simulink model "PenduloSimple"  (R2016a)
settings: Solver=VariableStepAuto  StartTime=0.0  StopTime=30  RelTol=1e-3
settings Model: Creator=i95sa  LastModifiedBy=i95sa

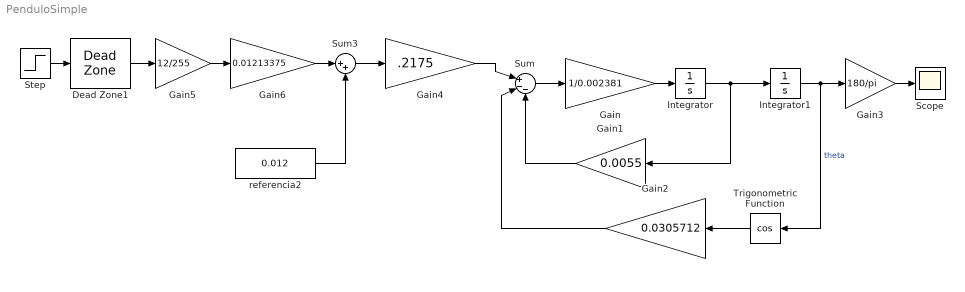
== system PenduloSimple ==
  Dead Zone1 : DeadZone  LowerValue=0  UpperValue=175  SaturateOnIntegerOverflow=on
  Gain : Gain  Gain=1/0.002381
  Gain1 : Gain  Gain=0.0055
  Gain2 : Gain  Gain=0.0305712
  Gain3 : Gain  Gain=180/pi
  Gain4 : Gain  Gain=.2175
  Gain5 : Gain  Gain=12/255
  Gain6 : Gain  Gain=0.01213375
  Integrator : Integrator
  Integrator1 : Integrator  InitialCondition=-0.6527531
  Scope : Scope
  Step : Step  Time=0  After=225  SampleTime=0
  Sum : Sum  Inputs=|+--
  Sum3 : Sum  Inputs=|++
  Trigonometric Function : Trigonometry  Operator=cos
  referencia2 : Constant  Value=0.012
  wires:
  Sum/1 -> Gain/1
  Gain/1 -> Integrator/1
  Integrator/1 -> Gain1/1, Integrator1/1
  Trigonometric Function/1 -> Gain2/1
  Gain1/1 -> Sum/3
  Integrator1/1 -> Gain3/1, Trigonometric Function/1  "theta"
  Gain2/1 -> Sum/2
  Gain3/1 -> Scope/1
  Gain4/1 -> Sum/1
  referencia2/1 -> Sum3/2
  Sum3/1 -> Gain4/1
  Step/1 -> Dead Zone1/1
  Gain5/1 -> Gain6/1
  Gain6/1 -> Sum3/1
  Dead Zone1/1 -> Gain5/1
